simulink model "HIL_comm"  (R2022a)
settings: Solver=FixedStepAuto  StartTime=0.0  StopTime=10.0  FixedStep=vdc_TimeStep  RelTol=1e-3
undefined symbols (not defined in the file): canChannel, param, param_vdc, vdc_TimeStep
libraries: canmsglib x9, canlib x4
settings Model: Creator=Usuario  LastModifiedBy=Usuario

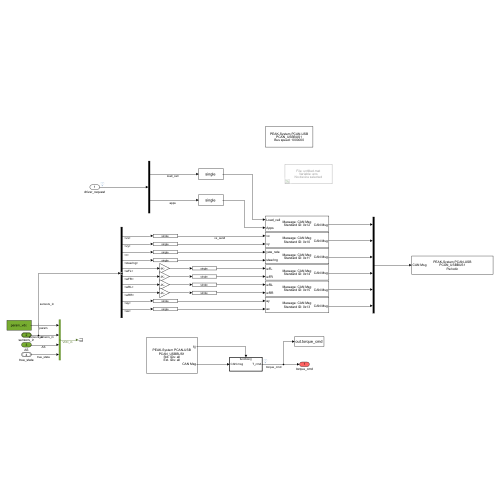
[thumbnail: Simulink's stored preview of the top-level diagram]
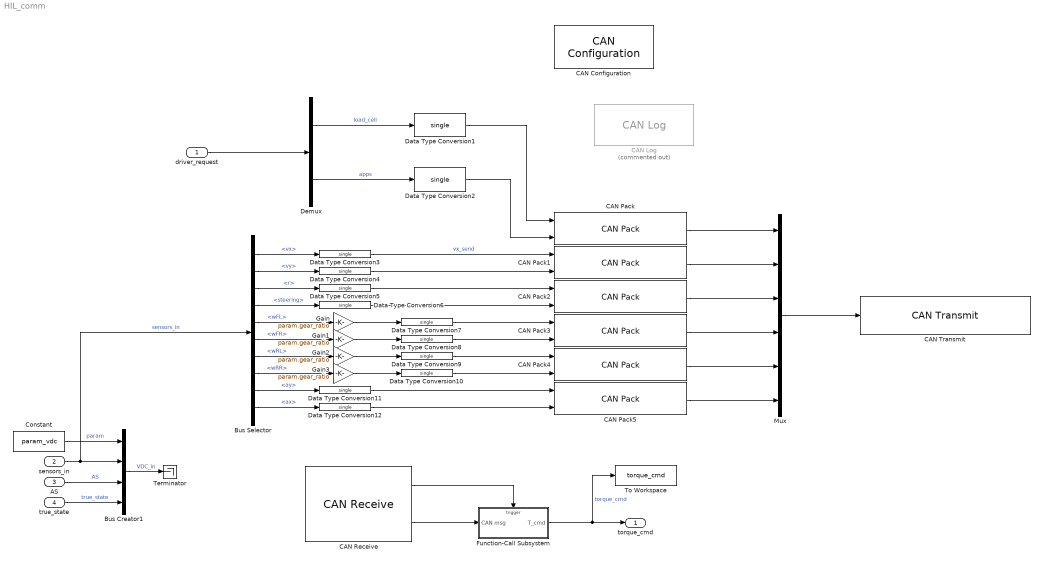
== system HIL_comm ==
  driver_request : Inport
  sensors_in : Inport  Port=2  OutDataTypeStr=Bus: sensorBus
  AS : Inport  Port=3
  true_state : Inport  Port=4  OutDataTypeStr=Bus: stateBus
  Bus Creator1 : BusCreator  Inputs=4
  Bus Selector : BusSelector  OutputSignals=gss.vx,gss.vy,gss.r,ext.steering,encoder.wFL,encoder.wFR,encoder.wRL,encoder.wRR,IMU.ay,IMU.ax
  CAN Configuration : canlib/CAN Configuration  BlockHandle=7588.0002  Device=PEAK-System PCAN-USB (PCAN_USBBUS1)  DeviceMenu=PEAK-System PCAN-USB (PCAN_USBBUS1)  ObjConstructor=canChannel('PEAK-System', 'PCAN_USBBUS1')  BusSpeed=1000000  EnableBitParameters=off  AckMode=Normal
      settings: SourceProductBaseCode=VN
  CAN Log : canlib/CAN Log  Commented=on  BlockHandle=7589.0002  FullPathFileName=untitled.mat  FileName=untitled.mat  VariableName=ans  MaxNumMessages=10000  LogFrom=CAN Bus  DeviceMenu=Select a device  Device=Select a device  ObjConstructor=Select a constructor  SampleTime=0.01
      settings: SourceProductBaseCode=VN
  CAN Pack : canmsglib/CAN Pack  MsgList=(none)  MsgName=CAN Msg  MsgIDType=Standard (11-bit identifier)  MsgIdentifier=0x12  MsgLength=8  Remote=off  ApplyMinMax=off  BusOutput=off  SignalInfo={ 'Load_cell', '0', '32', 'LE', 'single', 'Standard', '0', '1', '0', '-Inf', 'Inf'; 'Apps', '32', '32', 'LE', 'single', 'Standard', '0', '1', '0', '-Inf', 'Inf' }
      settings: SourceProductBaseCode=XP,ME,VN  DataFormat=manually specified signals
  CAN Pack1 : canmsglib/CAN Pack  MsgList=(none)  MsgName=CAN Msg  MsgIDType=Standard (11-bit identifier)  MsgIdentifier=0x10  MsgLength=8  Remote=off  ApplyMinMax=off  BusOutput=off  SignalInfo={ 'vx', '0', '32', 'LE', 'single', 'Standard', '0', '1', '0', '-Inf', 'Inf'; 'vy', '32', '32', 'LE', 'single', 'Standard', '0', '1', '0', '-Inf', 'Inf' }
      settings: SourceProductBaseCode=XP,ME,VN  DataFormat=manually specified signals
  CAN Pack2 : canmsglib/CAN Pack  MsgList=(none)  MsgName=CAN Msg  MsgIDType=Standard (11-bit identifier)  MsgIdentifier=0x11  MsgLength=8  Remote=off  ApplyMinMax=off  BusOutput=off  SignalInfo={ 'yaw_rate', '0', '32', 'LE', 'single', 'Standard', '0', '1', '0', '-Inf', 'Inf'; 'steering', '32', '32', 'LE', 'single', 'Standard', '0', '1', '0', '-Inf', 'Inf' }
      settings: SourceProductBaseCode=XP,ME,VN  DataFormat=manually specified signals
  CAN Pack3 : canmsglib/CAN Pack  MsgList=(none)  MsgName=CAN Msg  MsgIDType=Standard (11-bit identifier)  MsgIdentifier=0x14  MsgLength=8  Remote=off  ApplyMinMax=off  BusOutput=off  SignalInfo={ 'wFL', '0', '32', 'LE', 'single', 'Standard', '0', '1', '0', '-Inf', 'Inf'; 'wFR', '32', '32', 'LE', 'single', 'Standard', '0', '1', '0', '-Inf', 'Inf' }
      settings: SourceProductBaseCode=XP,ME,VN  DataFormat=manually specified signals
  CAN Pack4 : canmsglib/CAN Pack  MsgList=(none)  MsgName=CAN Msg  MsgIDType=Standard (11-bit identifier)  MsgIdentifier=0x15  MsgLength=8  Remote=off  ApplyMinMax=off  BusOutput=off  SignalInfo={ 'wRL', '0', '32', 'LE', 'single', 'Standard', '0', '1', '0', '-Inf', 'Inf'; 'wRR', '32', '32', 'LE', 'single', 'Standard', '0', '1', '0', '-Inf', 'Inf' }
      settings: SourceProductBaseCode=XP,ME,VN  DataFormat=manually specified signals
  CAN Pack5 : canmsglib/CAN Pack  MsgList=(none)  MsgName=CAN Msg  MsgIDType=Standard (11-bit identifier)  MsgIdentifier=0x13  MsgLength=8  Remote=off  ApplyMinMax=off  BusOutput=off  SignalInfo={ 'ay', '0', '32', 'LE', 'single', 'Standard', '0', '1', '0', '-Inf', 'Inf'; 'ax', '32', '32', 'LE', 'single', 'Standard', '0', '1', '0', '-Inf', 'Inf' }
      settings: SourceProductBaseCode=XP,ME,VN  DataFormat=manually specified signals
  CAN Receive : canlib/CAN Receive  BlockHandle=7614.0002  Device=PEAK-System PCAN-USB (PCAN_USBBUS1)  DeviceMenu=PEAK-System PCAN-USB (PCAN_USBBUS1)  ObjConstructor=canChannel('PEAK-System', 'PCAN_USBBUS1')  EnableStandardIDsFilter=off  StdIDsCombo=Allow all  StandardIDs=0  EnableExtendedIDsFilter=off  ExtIDsCombo=Allow all  ExtendedIDs=0  SampleTime=vdc_TimeStep  MsgsPerTimestep=all  InternalFilterUpdateStatus=on  BusOutput=off
      settings: SourceProductBaseCode=VN
  CAN Transmit : canlib/CAN Transmit  BlockHandle=7617.0002  Device=PEAK-System PCAN-USB (PCAN_USBBUS1)  DeviceMenu=PEAK-System PCAN-USB (PCAN_USBBUS1)  ObjConstructor=canChannel('PEAK-System', 'PCAN_USBBUS1')  EnableEventTransmit=off  EnablePeriodicTransmit=on  MessagePeriod=vdc_TimeStep
      settings: SourceProductBaseCode=VN
  Constant : Constant  Value=param_vdc  OutDataTypeStr=Bus: vdcBus
  Data Type Conversion{1..12} (12 alike) : DataTypeConversion  OutDataTypeStr=single  SaturateOnIntegerOverflow=off  RndMeth=Floor
  Demux : Demux  Outputs=2
  Function-Call Subsystem : Subsystem  TreatAsAtomicUnit=on
  Gain{,1..3} (4 alike) : Gain  Gain=param.gear_ratio
  Mux : Mux  Inputs=6
  Terminator : Terminator
  To Workspace : ToWorkspace  VariableName=torque_cmd  SaveFormat=Structure With Time  SampleTime=-1
  torque_cmd : Outport
  wires:
  Data Type Conversion1/1 -> CAN Pack/1
  true_state/1 -> Bus Creator1/4  "true_state"
  sensors_in/1 -> Bus Selector/1, Bus Creator1/2  "sensors_in"
  AS/1 -> Bus Creator1/3  "AS"
  Constant/1 -> Bus Creator1/1  "param"
  driver_request/1 -> Demux/1
  Demux/1 -> Data Type Conversion1/1  "load_cell"
  Data Type Conversion2/1 -> CAN Pack/2
  Demux/2 -> Data Type Conversion2/1  "apps"
  Bus Selector/1 -> Data Type Conversion3/1  "<vx>"
  Bus Selector/2 -> Data Type Conversion4/1  "<vy>"
  Bus Selector/3 -> Data Type Conversion5/1  "<r>"
  Bus Selector/10 -> Data Type Conversion12/1  "<ax>"
  Bus Selector/9 -> Data Type Conversion11/1  "<ay>"
  Bus Selector/8 -> Gain3/1  "<wRR>"
  Bus Selector/7 -> Gain2/1  "<wRL>"
  Bus Selector/6 -> Gain1/1  "<wFR>"
  Bus Selector/5 -> Gain/1  "<wFL>"
  Bus Selector/4 -> Data Type Conversion6/1  "<steering>"
  Data Type Conversion3/1 -> CAN Pack1/1  "vx_send"
  Data Type Conversion4/1 -> CAN Pack1/2
  Data Type Conversion5/1 -> CAN Pack2/1
  Data Type Conversion6/1 -> CAN Pack2/2
  Data Type Conversion7/1 -> CAN Pack3/1
  Data Type Conversion8/1 -> CAN Pack3/2
  Data Type Conversion9/1 -> CAN Pack4/1
  Data Type Conversion10/1 -> CAN Pack4/2
  Data Type Conversion11/1 -> CAN Pack5/1
  Data Type Conversion12/1 -> CAN Pack5/2
  Gain/1 -> Data Type Conversion7/1
  Gain1/1 -> Data Type Conversion8/1
  Gain2/1 -> Data Type Conversion9/1
  Gain3/1 -> Data Type Conversion10/1
  Bus Creator1/1 -> Terminator/1  "VDC_in"
  CAN Receive/1 -> Function-Call Subsystem/Trigger
  CAN Receive/2 -> Function-Call Subsystem/1(CAN msg)
  Function-Call Subsystem/1(T_cmd) -> To Workspace/1, torque_cmd/1  "torque_cmd"
  CAN Pack/1 -> Mux/1
  Mux/1 -> CAN Transmit/1
  CAN Pack5/1 -> Mux/6
  CAN Pack4/1 -> Mux/5
  CAN Pack3/1 -> Mux/4
  CAN Pack2/1 -> Mux/3
  CAN Pack1/1 -> Mux/2

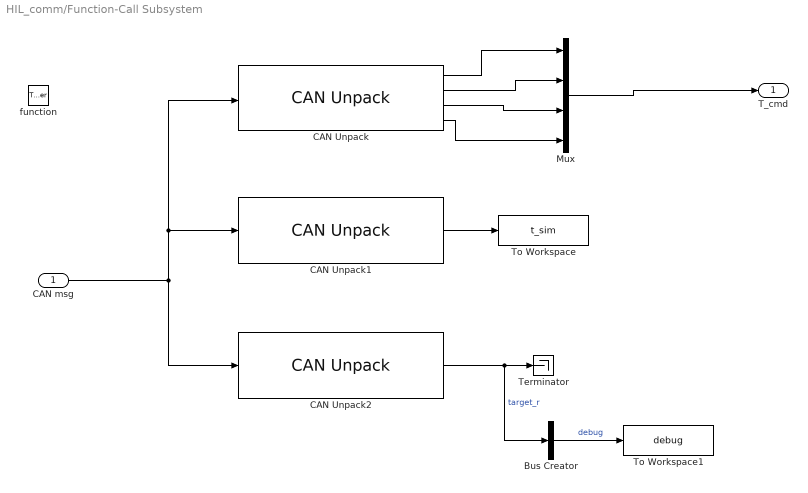
== system HIL_comm/Function-Call Subsystem ==
  CAN msg : Inport
  function : TriggerPort  TriggerType=function-call  VariantControl=(inherit)
  Bus Creator : BusCreator  Inputs=1
  CAN Unpack : canmsglib/CAN Unpack  MsgList=(none)  MsgName=Prueba  MsgIDType=Standard (11-bit identifier)  MsgIdentifier=0x100  MsgLength=8  SignalInfo={ 'Torque_FL', '0', '16', 'LE', 'signed', 'Standard', '0', '0.01', '0', '-Inf', 'Inf'; 'Torque_FR', '16', '16', 'LE', 'signed', 'Standard', '0', '0.01', '0', '-Inf', 'Inf'; 'Torque_RL', '32', '16', 'LE', 'signed', 'Standard', '0', '0.01', '0', '-Inf', 'Inf'; 'Torque_RR', '48', '16', 'LE', 'signed', 'Standard', '0', '0.01', '0', '-Inf', 'Inf' }  IDPort=off  TimestampPort=off  ErrorPort=off  RemotePort=off  LengthPort=off  StatusPort=off  ApplyMinMax=off
      settings: SourceProductBaseCode=XP,ME,VN
  CAN Unpack1 : canmsglib/CAN Unpack  MsgList=(none)  MsgName=Prueba  MsgIDType=Standard (11-bit identifier)  MsgIdentifier=0x101  MsgLength=2  SignalInfo={ 'T_sim', '0', '16', 'LE', 'signed', 'Standard', '0', '0.0001', '0', '-Inf', 'Inf' }  IDPort=off  TimestampPort=off  ErrorPort=off  RemotePort=off  LengthPort=off  StatusPort=off  ApplyMinMax=off
      settings: SourceProductBaseCode=XP,ME,VN
  CAN Unpack2 : canmsglib/CAN Unpack  MsgList=(none)  MsgName=Prueba  MsgIDType=Standard (11-bit identifier)  MsgIdentifier=0x102  MsgLength=2  SignalInfo={ 'target_r', '0', '16', 'LE', 'signed', 'Standard', '0', '0.01', '0', '-Inf', 'Inf' }  IDPort=off  TimestampPort=off  ErrorPort=off  RemotePort=off  LengthPort=off  StatusPort=off  ApplyMinMax=off
      settings: SourceProductBaseCode=XP,ME,VN
  Mux : Mux
  Terminator : Terminator
  To Workspace : ToWorkspace  VariableName=t_sim  SaveFormat=Structure With Time  SampleTime=-1
  To Workspace1 : ToWorkspace  VariableName=debug  SaveFormat=Structure With Time  SampleTime=-1
  T_cmd : Outport
  wires:
  CAN Unpack/1 -> Mux/1
  CAN Unpack/2 -> Mux/2
  Mux/1 -> T_cmd/1
  CAN Unpack/3 -> Mux/3
  CAN Unpack/4 -> Mux/4
  CAN Unpack1/1 -> To Workspace/1
  CAN Unpack2/1 -> Bus Creator/1, Terminator/1  "target_r"
  CAN msg/1 -> CAN Unpack1/1, CAN Unpack/1, CAN Unpack2/1
  Bus Creator/1 -> To Workspace1/1  "debug"
